simulink subsystem "Magnetometer"  (R2021a)
settings: Solver=VariableStepAuto  StartTime=0.0  StopTime=10.0  RelTol=1e-3
libraries: simulink x4, sharedtransform x1
settings Model: Creator=jmher  LastModifiedBy=jmher

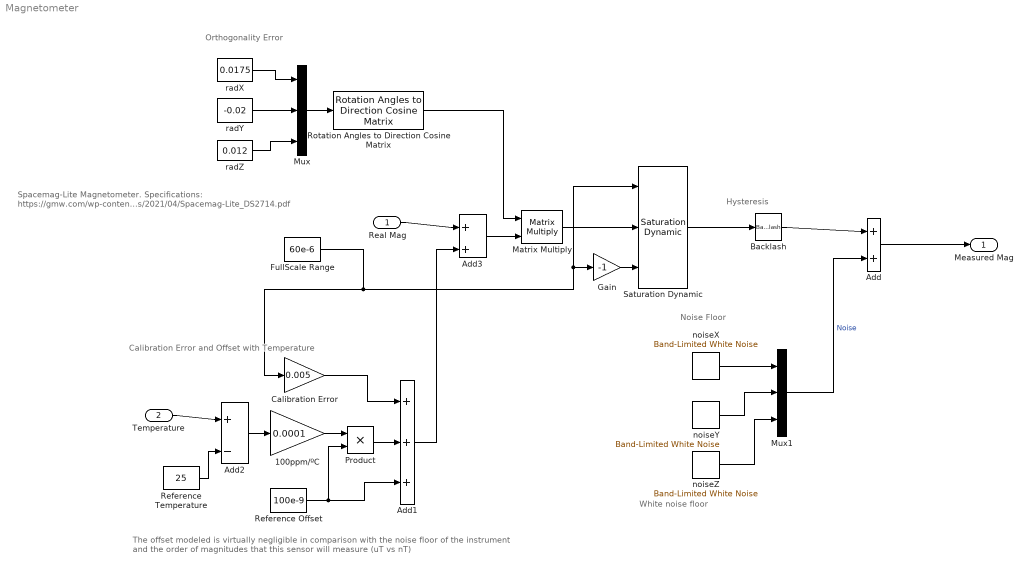
== system Magnetometer ==
  note: Hysteresis
  note: Noise Floor
  note: Orthogonality Error
  note: Calibration Error and Offset
      | with Temperature
  note: Spacemag-Lite Magnetometer.
      |
      | Specifications: https://gmw.com/wp-content/uploads/2021/04/Spacemag-Lite_DS2714.pdf
  note: White noise floor
  note: The offset modeled is virtually negligible in comparison with the noise floor of the instrument and the order of magnitudes that this sensor will measure (uT vs nT)
  Real Mag : Inport
  Temperature : Inport  Port=2
  100ppm/ºC : Gain  Gain=0.0001
  Add : Sum  Inputs=+|+
  Add1 : Sum  Inputs=+|+|+
  Add2 : Sum  Inputs=+|-
  Add3 : Sum  Inputs=+|+
  Backlash : Backlash  BacklashWidth=hyst  InputProcessing=Columns as channels (frame based)
  Calibration Error : Gain  Gain=0.005
  FullScale Range : Constant  Value=60e-6
  Gain : Gain  Gain=-1
  Matrix Multiply : Product  Multiplication=Matrix(*)
  Mux : Mux  Inputs=3
  Mux1 : Mux  Inputs=3
  Product : Product
  Reference Offset : Constant  Value=100e-9
  Reference Temperature : Constant  Value=25
  Rotation Angles to Direction Cosine Matrix : sharedtransform/Rotation Angles to Direction Cosine Matrix  rotationOrder=ZYX  aMode=aMode
      settings: SourceProductBaseCode=AE,PW,DR,MT,UV,VE
  Saturation Dynamic : simulink/Discontinuities/Saturation Dynamic  OutMin=[]  OutMax=[]  OutDataTypeStr=Inherit: Same as second input  OutDataType=fixdt(1, 16)  OutScaling=2^-10  RndMeth=Round  DoSatur=off
  noiseX : simulink/Sources/Band-Limited White Noise  Cov=noiseDens  Ts=0.001  seed=[47561]
  noiseY : simulink/Sources/Band-Limited White Noise  Cov=noiseDens  Ts=0.001  seed=[238641]
  noiseZ : simulink/Sources/Band-Limited White Noise  Cov=noiseDens  Ts=0.001  seed=[23341]
  radX : Constant  Value=0.0175
  radY : Constant  Value=-0.02
  radZ : Constant  Value=0.012
  Measured Mag : Outport
  wires:
  FullScale Range/1 -> Calibration Error/1, Gain/1, Saturation Dynamic/1
  Gain/1 -> Saturation Dynamic/3
  Mux/1 -> Rotation Angles to Direction Cosine Matrix/1
  radX/1 -> Mux/1
  radY/1 -> Mux/2
  radZ/1 -> Mux/3
  Rotation Angles to Direction Cosine Matrix/1 -> Matrix Multiply/1
  noiseX/1 -> Mux1/1
  noiseY/1 -> Mux1/2
  noiseZ/1 -> Mux1/3
  Add/1 -> Measured Mag/1
  Backlash/1 -> Add/1
  Mux1/1 -> Add/2  "Noise"
  Calibration Error/1 -> Add1/1
  Add2/1 -> 100ppm/ºC/1
  Temperature/1 -> Add2/1
  Reference Temperature/1 -> Add2/2
  Reference Offset/1 -> Add1/3, Product/2
  Add1/1 -> Add3/2
  Real Mag/1 -> Add3/1
  Add3/1 -> Matrix Multiply/2
  Matrix Multiply/1 -> Saturation Dynamic/2
  Saturation Dynamic/1 -> Backlash/1
  100ppm/ºC/1 -> Product/1
  Product/1 -> Add1/2
